simulink model "motor_3"  (R2023a)
settings: Solver=ode15s  StartTime=0.0  StopTime=sim_end_time  MaxStep=0.0001  RelTol=1e-3
values from neighbouring files (symbols this model uses):
  alpha_cu = 3.9 *10^-3    (= 0.0039)    [BLDC_Motor_params_03.m]    (also in DC_Motor_params_01.m; DC_Motor_params_02.m; DC_Motor_params_04.m; DC_Motor_params_05.m)
  b_m3 = .001    (= 0.001)    [BLDC_Motor_params_03.m]
  C_t3 = 50    [BLDC_Motor_params_03.m]
  ENABLE_SATURATIONS = 1    [run_flags.m]
  J_eq3 = J_3 + 1/8 * m_3 * d_3^2 / r_3^2    [BLDC_Motor_params_03.m]
  K_d3 = 0    [PID_tuning.m]
  k_e3 = 0.3    [BLDC_Motor_params_03.m]
  K_i3 = 0.4131    [PID_tuning.m]
  K_p3 = 0    [PID_tuning.m]
  k_t3 = 0.3    [BLDC_Motor_params_03.m]
  L_a3 = 5*10^-3    (= 0.005)    [BLDC_Motor_params_03.m]
  r_3 = 2    [BLDC_Motor_params_03.m]
  r_a3_20 = 0.35    [BLDC_Motor_params_03.m]
  res_term_3 = 0.1    [BLDC_Motor_params_03.m]
  voltage_3 = 220    [BLDC_Motor_params_03.m]
  w_m3_0 = ans.simulationOut.Data(end,1)    [use_solo_motor_3.m]
settings Model: Creator=Usuario  LastModifiedBy=Usuario

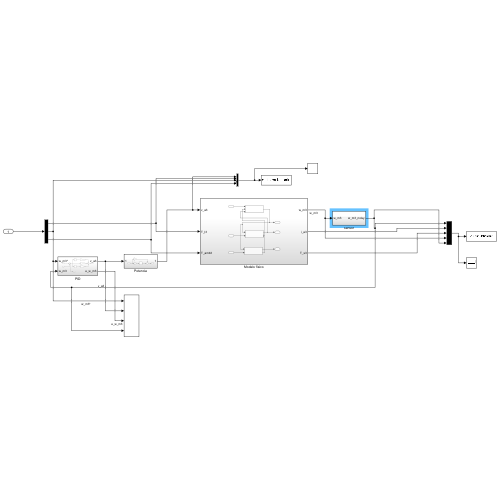
[thumbnail: Simulink's stored preview of the top-level diagram]
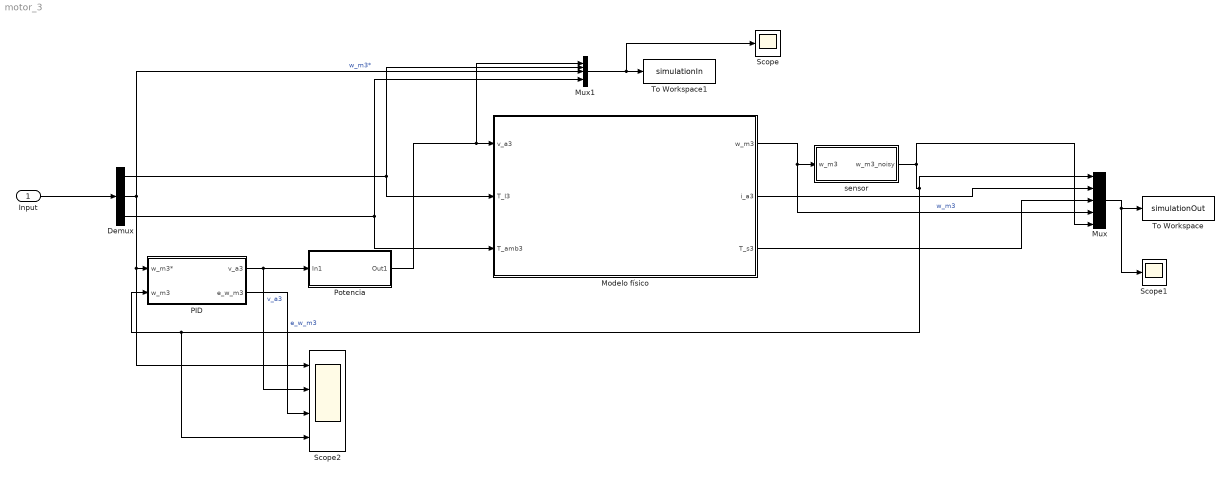
== system motor_3 ==
  Input : Inport
  Demux : Demux  Outputs=3
  Modelo físico : Subsystem
  Mux : Mux  Inputs=5
  Mux1 : Mux  Inputs=5
  PID : Subsystem
  Potencia : Subsystem
  Scope : Scope
  Scope1 : Scope
  Scope2 : Scope  NumInputPorts=4
  To Workspace : ToWorkspace  VariableName=simulationOut  SaveFormat=Timeseries  SampleTime=-1
  To Workspace1 : ToWorkspace  VariableName=simulationIn  SaveFormat=Timeseries  SampleTime=-1
  sensor : Subsystem
  wires:
  PID/2(e_w_m3) -> Scope2/3  "e_w_m3"
  Demux/1 -> Modelo físico/2(T_l3), Mux1/2
  Demux/2 -> Scope2/1, PID/1(w_m3*), Mux1/3  "w_m3*"
  Modelo físico/1(w_m3) -> Mux/4, sensor/1(w_m3)  "w_m3"
  Input/1 -> Demux/1
  Modelo físico/2(i_a3) -> Mux/2
  Mux1/1 -> Scope/1, To Workspace1/1
  Demux/3 -> Modelo físico/3(T_amb3), Mux1/5
  Mux/1 -> Scope1/1, To Workspace/1
  Modelo físico/3(T_s3) -> Mux/3
  PID/1(v_a3) -> Scope2/2, Potencia/1(In1)  "v_a3"
  Potencia/1(Out1) -> Modelo físico/1(v_a3), Mux1/1
  sensor/1(w_m3_noisy) -> Mux/5, Scope2/4, PID/2(w_m3), Mux/1

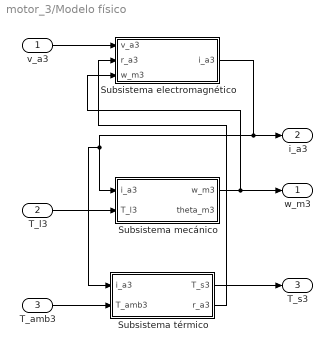
== system motor_3/Modelo físico ==
  v_a3 : Inport
  T_l3 : Inport  Port=2
  T_amb3 : Inport  Port=3
  Subsistema electromagnético : Subsystem
  Subsistema mecánico : Subsystem
  Subsistema térmico : Subsystem
  w_m3 : Outport
  i_a3 : Outport  Port=2
  T_s3 : Outport  Port=3
  wires:
  Subsistema electromagnético/1(i_a3) -> Subsistema térmico/1(i_a3), Subsistema mecánico/1(i_a3), i_a3/1
  v_a3/1 -> Subsistema electromagnético/1(v_a3)
  T_l3/1 -> Subsistema mecánico/2(T_l3)
  Subsistema mecánico/1(w_m3) -> w_m3/1, Subsistema electromagnético/3(w_m3)
  T_amb3/1 -> Subsistema térmico/2(T_amb3)
  Subsistema térmico/1(T_s3) -> T_s3/1
  Subsistema térmico/2(r_a3) -> Subsistema electromagnético/2(r_a3)

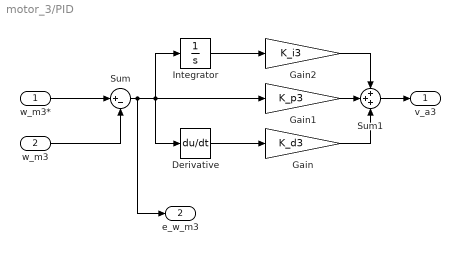
== system motor_3/PID ==
  w_m3* : Inport
  w_m3 : Inport  Port=2
  Derivative : Derivative
  Gain : Gain  Gain=K_d3
  Gain1 : Gain  Gain=K_p3
  Gain2 : Gain  Gain=K_i3
  Integrator : Integrator
  Sum : Sum  Inputs=|+-
  Sum1 : Sum  Inputs=+++
  v_a3 : Outport
  e_w_m3 : Outport  Port=2
  wires:
  w_m3*/1 -> Sum/1
  w_m3/1 -> Sum/2
  Sum/1 -> e_w_m3/1, Integrator/1, Gain1/1, Derivative/1
  Integrator/1 -> Gain2/1
  Derivative/1 -> Gain/1
  Gain1/1 -> Sum1/2
  Gain2/1 -> Sum1/1
  Sum1/1 -> v_a3/1
  Gain/1 -> Sum1/3

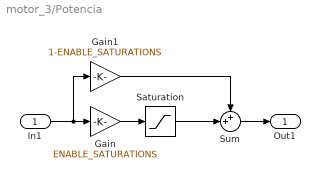
== system motor_3/Potencia ==
  In1 : Inport
  Gain : Gain  Gain=ENABLE_SATURATIONS
  Gain1 : Gain  Gain=1-ENABLE_SATURATIONS
  Saturation : Saturate  UpperLimit=+voltage_3  LowerLimit=-voltage_3
  Sum : Sum  Inputs=++|
  Out1 : Outport
  wires:
  In1/1 -> Gain1/1, Gain/1
  Saturation/1 -> Sum/2
  Gain/1 -> Saturation/1
  Sum/1 -> Out1/1
  Gain1/1 -> Sum/1

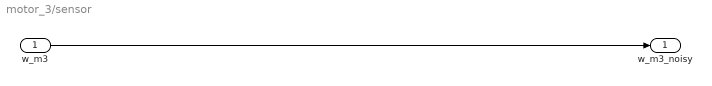
== system motor_3/sensor ==
  w_m3 : Inport
  w_m3_noisy : Outport
  wires:
  w_m3/1 -> w_m3_noisy/1

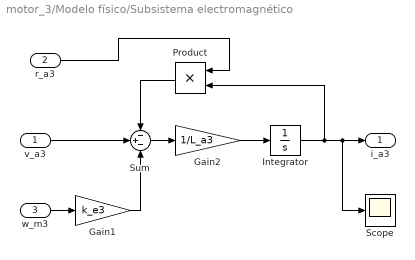
== system motor_3/Modelo físico/Subsistema electromagnético ==
  v_a3 : Inport
  r_a3 : Inport  Port=2
  w_m3 : Inport  Port=3
  Gain1 : Gain  Gain=k_e3
  Gain2 : Gain  Gain=1/L_a3
  Integrator : Integrator
  Product : Product
  Scope : Scope
  Sum : Sum  Inputs=-+-
  i_a3 : Outport
  wires:
  v_a3/1 -> Sum/2
  Integrator/1 -> Product/2, Scope/1, i_a3/1
  Product/1 -> Sum/1
  w_m3/1 -> Gain1/1
  Gain1/1 -> Sum/3
  Sum/1 -> Gain2/1
  Gain2/1 -> Integrator/1
  r_a3/1 -> Product/1

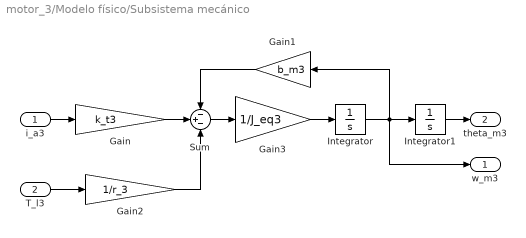
== system motor_3/Modelo físico/Subsistema mecánico ==
  i_a3 : Inport
  T_l3 : Inport  Port=2
  Gain : Gain  Gain=k_t3
  Gain1 : Gain  Gain=b_m3
  Gain2 : Gain  Gain=1/r_3
  Gain3 : Gain  Gain=1/J_eq3
  Integrator : Integrator  InitialCondition=w_m3_0
  Integrator1 : Integrator
  Sum : Sum  Inputs=-+-
  w_m3 : Outport
  theta_m3 : Outport  Port=2
  wires:
  i_a3/1 -> Gain/1
  Gain/1 -> Sum/2
  Integrator/1 -> w_m3/1, Gain1/1, Integrator1/1
  Gain1/1 -> Sum/1
  T_l3/1 -> Gain2/1
  Gain3/1 -> Integrator/1
  Sum/1 -> Gain3/1
  Integrator1/1 -> theta_m3/1
  Gain2/1 -> Sum/3

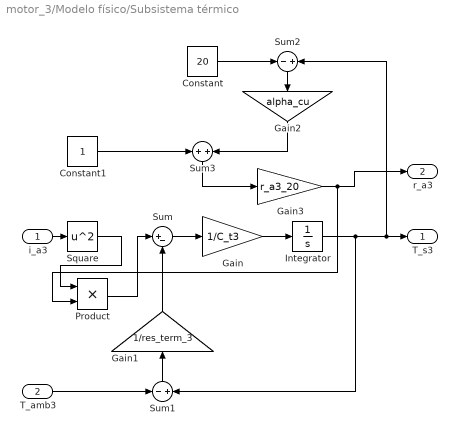
== system motor_3/Modelo físico/Subsistema térmico ==
  i_a3 : Inport
  T_amb3 : Inport  Port=2
  Constant : Constant  Value=20
  Constant1 : Constant
  Gain : Gain  Gain=1/C_t3
  Gain1 : Gain  Gain=1/res_term_3
  Gain2 : Gain  Gain=alpha_cu
  Gain3 : Gain  Gain=r_a3_20
  Integrator : Integrator
  Product : Product
  Square : Math  Operator=square
  Sum : Sum  Inputs=|+-
  Sum1 : Sum  Inputs=-|+
  Sum2 : Sum  Inputs=-|+
  Sum3 : Sum  Inputs=+|+
  T_s3 : Outport
  r_a3 : Outport  Port=2
  wires:
  i_a3/1 -> Square/1
  Sum3/1 -> Gain3/1
  Gain2/1 -> Sum3/2
  Square/1 -> Product/1
  Gain3/1 -> Product/2, r_a3/1
  Sum2/1 -> Gain2/1
  T_amb3/1 -> Sum1/1
  Constant1/1 -> Sum3/1
  Gain/1 -> Integrator/1
  Sum/1 -> Gain/1
  Integrator/1 -> Sum1/2, Sum2/2, T_s3/1
  Constant/1 -> Sum2/1
  Sum1/1 -> Gain1/1
  Gain1/1 -> Sum/2
  Product/1 -> Sum/1
